simulink model "DC_Parameter_estimation_DREM"  (R2022b)
settings: Solver=VariableStepAuto  StartTime=0.0  StopTime=20  RelTol=1e-3
undefined symbols (not defined in the file): alpha_1, alpha_2, alpha_3
settings Model: Creator=asala  LastModifiedBy=asala

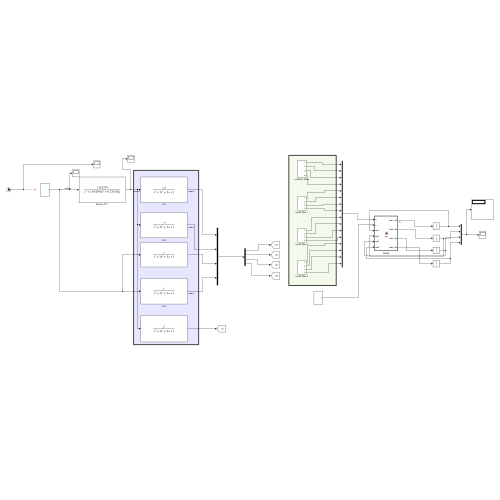
[thumbnail: Simulink's stored preview of the top-level diagram]
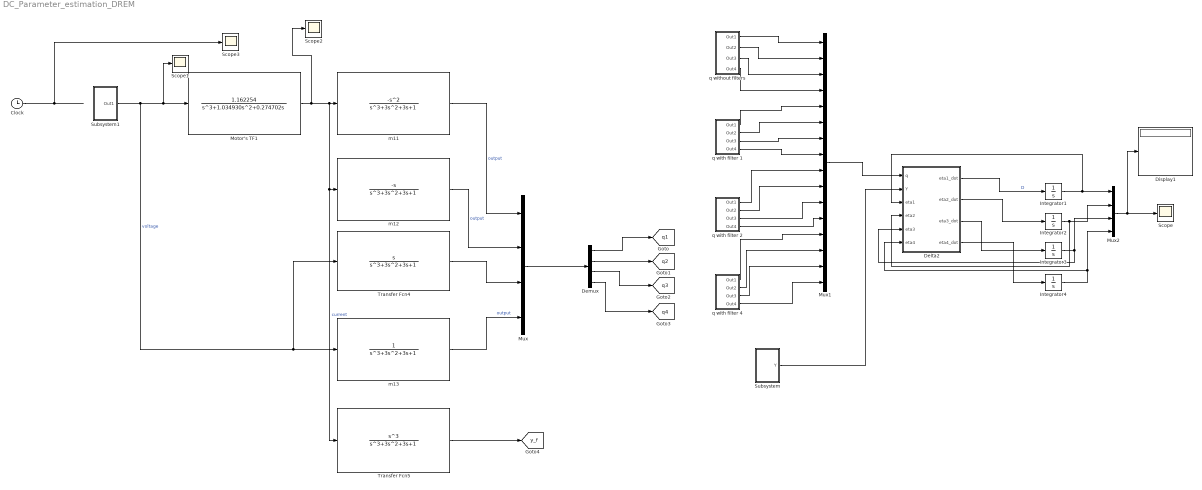
== system DC_Parameter_estimation_DREM ==
  Clock : Clock
  Delta2 : MATLAB Function  TreatAsAtomicUnit=on
  Demux : Demux
  Display1 : Display
  Integrator{1..4} (4 alike) : Integrator
  Motor's TF1 : TransferFcn  Numerator=[1.162254]  Denominator=[1 1.034930 0.274702 0]
  Mux : Mux
  Mux1 : Mux  Inputs=16
  Mux2 : Mux
  Scope{,1..3} (4 alike) : Scope
  Subsystem : Subsystem
  Subsystem1 : Subsystem
  Transfer Fcn4 : TransferFcn  Numerator=[0 1 0]  Denominator=[1, 3, 3, 1]
  Transfer Fcn5 : TransferFcn  Numerator=[1 0 0 0]  Denominator=[1, 3, 3, 1]
  m11 : TransferFcn  Numerator=[-1 0 0]  Denominator=[1, 3, 3, 1]
  m12 : TransferFcn  Numerator=[0 -1 0]  Denominator=[1, 3, 3, 1]
  m13 : TransferFcn  Numerator=[0 0 1]  Denominator=[1, 3, 3, 1]
  q with filter 1 : Subsystem
  q with filter 2 : Subsystem
  q with filter 4 : Subsystem
  q without filters : Subsystem
  tag scope: q1=global, q2=global, q3=global, q4=global, y_f=global
  wires:
  Subsystem1/1(Out1) -> Transfer Fcn4/1, m13/1, Scope1/1, Motor's TF1/1  "voltage"
  Clock/1 -> Scope3/1
  Motor's TF1/1 -> Scope2/1, Transfer Fcn5/1, m12/1, m11/1  "current"
  Demux/3 -> [q3]
  Demux/4 -> [q4]
  Demux/2 -> [q2]
  Demux/1 -> [q1]
  m11/1 -> Mux/1  "output"
  m12/1 -> Mux/2  "output"
  Transfer Fcn4/1 -> Mux/3
  m13/1 -> Mux/4  "output"
  Transfer Fcn5/1 -> [y_f]
  Mux/1 -> Demux/1
  q without filters/1(Out1) -> Mux1/1
  q without filters/2(Out2) -> Mux1/2
  q without filters/3(Out3) -> Mux1/3
  q without filters/4(Out4) -> Mux1/4
  q with filter 1/1(Out1) -> Mux1/5
  q with filter 1/2(Out2) -> Mux1/6
  q with filter 1/3(Out3) -> Mux1/7
  q with filter 1/4(Out4) -> Mux1/8
  q with filter 2/1(Out1) -> Mux1/9
  q with filter 2/2(Out2) -> Mux1/10
  q with filter 2/3(Out3) -> Mux1/11
  q with filter 2/4(Out4) -> Mux1/12
  q with filter 4/1(Out1) -> Mux1/13
  q with filter 4/2(Out2) -> Mux1/14
  q with filter 4/3(Out3) -> Mux1/15
  q with filter 4/4(Out4) -> Mux1/16
  Integrator1/1 -> Delta2/3(eta1), Mux2/1
  Delta2/1(eta1_dot) -> Integrator1/1  "D"
  Delta2/2(eta2_dot) -> Integrator2/1
  Delta2/3(eta3_dot) -> Integrator3/1
  Delta2/4(eta4_dot) -> Integrator4/1
  Integrator4/1 -> Delta2/6(eta4), Mux2/4
  Integrator2/1 -> Delta2/4(eta2), Mux2/2
  Integrator3/1 -> Mux2/3, Delta2/5(eta3)
  Mux1/1 -> Delta2/1(q)
  Subsystem/1(Y) -> Delta2/2(Y)
  Mux2/1 -> Scope/1, Display1/1

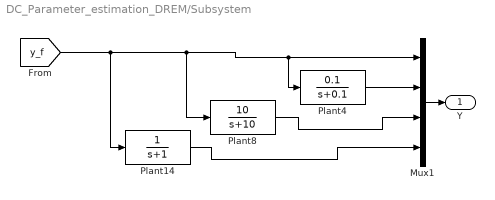
== system DC_Parameter_estimation_DREM/Subsystem ==
  Mux1 : Mux
  Plant14 : TransferFcn  Denominator=[1 1]
  Plant4 : TransferFcn  Numerator=[0.1]  Denominator=[1 0.1]
  Plant8 : TransferFcn  Numerator=[10]  Denominator=[1 10]
  Y : Outport  VectorParamsAs1DForOutWhenUnconnected=off
  wires:
  Mux1/1 -> Y/1
  [y_f] -> Plant14/1, Plant8/1, Plant4/1, Mux1/1
  Plant4/1 -> Mux1/2
  Plant14/1 -> Mux1/4
  Plant8/1 -> Mux1/3

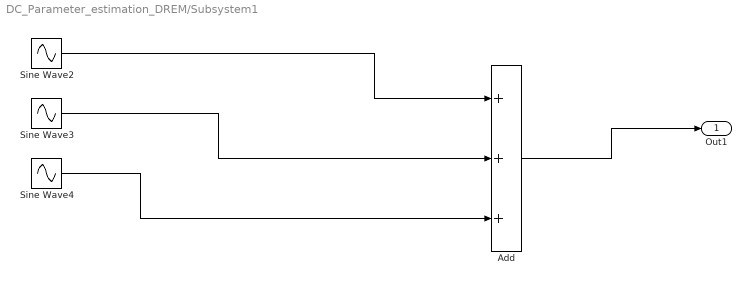
== system DC_Parameter_estimation_DREM/Subsystem1 ==
  Add : Sum  Inputs=+++
  Sine Wave2 : Sin  Amplitude=5  Frequency=2  SampleTime=0
  Sine Wave3 : Sin  Amplitude=2  Frequency=3  SampleTime=0
  Sine Wave4 : Sin  Amplitude=4  SampleTime=0
  Out1 : Outport  VectorParamsAs1DForOutWhenUnconnected=off
  wires:
  Add/1 -> Out1/1
  Sine Wave2/1 -> Add/1
  Sine Wave3/1 -> Add/2
  Sine Wave4/1 -> Add/3

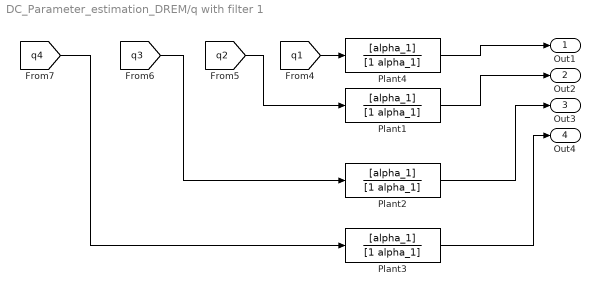
== system DC_Parameter_estimation_DREM/q with filter 1 ==
  Plant{1..4} (4 alike) : TransferFcn  Numerator=[alpha_1]  Denominator=[1 alpha_1]
  Out1 : Outport  VectorParamsAs1DForOutWhenUnconnected=off
  Out2 : Outport  Port=2  VectorParamsAs1DForOutWhenUnconnected=off
  Out3 : Outport  Port=3  VectorParamsAs1DForOutWhenUnconnected=off
  Out4 : Outport  Port=4  VectorParamsAs1DForOutWhenUnconnected=off
  wires:
  [q1] -> Plant4/1
  [q4] -> Plant3/1
  [q3] -> Plant2/1
  Plant2/1 -> Out3/1
  Plant4/1 -> Out1/1
  Plant3/1 -> Out4/1
  [q2] -> Plant1/1
  Plant1/1 -> Out2/1

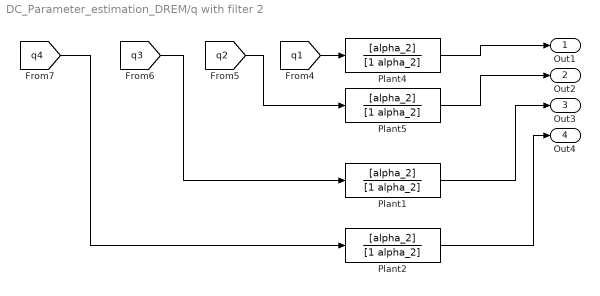
== system DC_Parameter_estimation_DREM/q with filter 2 ==
  Plant{1..2,4..5} (4 alike) : TransferFcn  Numerator=[alpha_2]  Denominator=[1 alpha_2]
  Out1 : Outport  VectorParamsAs1DForOutWhenUnconnected=off
  Out2 : Outport  Port=2  VectorParamsAs1DForOutWhenUnconnected=off
  Out3 : Outport  Port=3  VectorParamsAs1DForOutWhenUnconnected=off
  Out4 : Outport  Port=4  VectorParamsAs1DForOutWhenUnconnected=off
  wires:
  Plant5/1 -> Out2/1
  [q2] -> Plant5/1
  Plant2/1 -> Out4/1
  Plant4/1 -> Out1/1
  Plant1/1 -> Out3/1
  [q3] -> Plant1/1
  [q4] -> Plant2/1
  [q1] -> Plant4/1

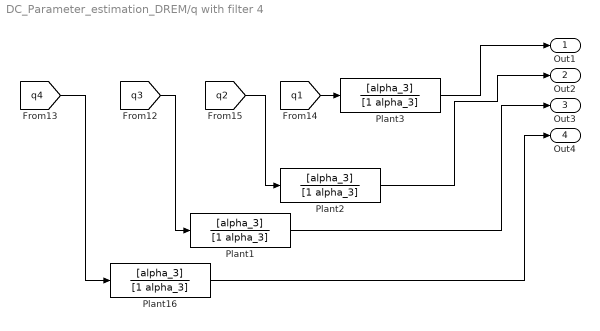
== system DC_Parameter_estimation_DREM/q with filter 4 ==
  Plant{1..3,16} (4 alike) : TransferFcn  Numerator=[alpha_3]  Denominator=[1 alpha_3]
  Out1 : Outport  VectorParamsAs1DForOutWhenUnconnected=off
  Out2 : Outport  Port=2  VectorParamsAs1DForOutWhenUnconnected=off
  Out3 : Outport  Port=3  VectorParamsAs1DForOutWhenUnconnected=off
  Out4 : Outport  Port=4  VectorParamsAs1DForOutWhenUnconnected=off
  wires:
  [q1] -> Plant3/1
  Plant1/1 -> Out3/1
  Plant2/1 -> Out2/1
  [q2] -> Plant2/1
  Plant16/1 -> Out4/1
  Plant3/1 -> Out1/1
  [q4] -> Plant16/1
  [q3] -> Plant1/1

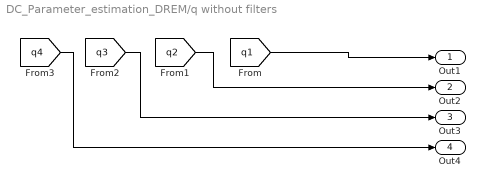
== system DC_Parameter_estimation_DREM/q without filters ==
  Out1 : Outport  VectorParamsAs1DForOutWhenUnconnected=off
  Out2 : Outport  Port=2  VectorParamsAs1DForOutWhenUnconnected=off
  Out3 : Outport  Port=3  VectorParamsAs1DForOutWhenUnconnected=off
  Out4 : Outport  Port=4  VectorParamsAs1DForOutWhenUnconnected=off
  wires:
  [q2] -> Out2/1
  [q4] -> Out4/1
  [q3] -> Out3/1
  [q1] -> Out1/1

== matlab function DC_Parameter_estimation_DREM/Delta2 ==
  data: q input; eta1_dot output; Y input; eta1 input; eta2 input; eta3 input; eta4 input; eta2_dot output; eta3_dot output; eta4_dot output
function [eta1_dot, eta2_dot, eta3_dot, eta4_dot] = fcn(q, Y, eta1, eta2, eta3, eta4)
gamma1=1000;
gamma2=1000;
gamma3=1000;
gamma4=1000;

q11=q(1);
q12=q(2);
q13=q(3);
q14=q(4);
q21=q(5);
q22=q(6);
q23=q(7);
q24=q(8);
q31=q(9);
q32=q(10);
q33=q(11);
q34=q(12);
q41=q(13);
q42=q(14);
q43=q(15);
q44=q(16);

y1=Y(1);
y2=Y(2);
y3=Y(3);
y4=Y(4);

zeta1= y3*(q12*q23*q44 - q12*q24*q43 - q13*q22*q44 + q13*q24*q42 + q14*q22*q43 - q14*q23*q42) - y4*(q12*q23*q34 - q12*q24*q33 - q13*q22*q34 + q13*q24*q32 + q14*q22*q33 - q14*q23*q32) - y2*(q12*q33*q44 - q12*q34*q43 - q13*q32*q44 + q13*q34*q42 + q14*q32*q43 - q14*q33*q42) + y1*(q22*q33*q44 - q22*q34*q43 - q23*q32*q44 + q23*q34*q42 + q24*q32*q43 - q24*q33*q42);
zeta2= y4*(q11*q23*q34 - q11*q24*q33 - q13*q21*q34 + q13*q24*q31 + q14*q21*q33 - q14*q23*q31) - y3*(q11*q23*q44 - q11*q24*q43 - q13*q21*q44 + q13*q24*q41 + q14*q21*q43 - q14*q23*q41) + y2*(q11*q33*q44 - q11*q34*q43 - q13*q31*q44 + q13*q34*q41 + q14*q31*q43 - q14*q33*q41) - y1*(q21*q33*q44 - q21*q34*q43 - q23*q31*q44 + q23*q34*q41 + q24*q31*q43 - q24*q33*q41);
zeta3= y3*(q11*q22*q44 - q11*q24*q42 - q12*q21*q44 + q12*q24*q41 + q14*q21*q42 - q14*q22*q41) - y4*(q11*q22*q34 - q11*q24*q32 - q12*q21*q34 + q12*q24*q31 + q14*q21*q32 - q14*q22*q31) - y2*(q11*q32*q44 - q11*q34*q42 - q12*q31*q44 + q12*q34*q41 + q14*q31*q42 - q14*q32*q41) + y1*(q21*q32*q44 - q21*q34*q42 - q22*q31*q44 + q22*q34*q41 + q24*q31*q42 - q24*q32*q41);
zeta4= y4*(q11*q22*q33 - q11*q23*q32 - q12*q21*q33 + q12*q23*q31 + q13*q21*q32 - q13*q22*q31) - y3*(q11*q22*q43 - q11*q23*q42 - q12*q21*q43 + q12*q23*q41 + q13*q21*q42 - q13*q22*q41) + y2*(q11*q32*q43 - q11*q33*q42 - q12*q31*q43 + q12*q33*q41 + q13*q31*q42 - q13*q32*q41) - y1*(q21*q32*q43 - q21*q33*q42 - q22*q31*q43 + q22*q33*q41 + q23*q31*q42 - q23*q32*q41);



phi=q11*q22*q33*q44 - q11*q22*q34*q43 - q11*q23*q32*q44 + q11*q23*q34*q42 + q11*q24*q32*q43 - q11*q24*q33*q42 - q12*q21*q33*q44 + q12*q21*q34*q43 + q12*q23*q31*q44 - q12*q23*q34*q41 - q12*q24*q31*q43 + q12*q24*q33*q41 + q13*q21*q32*q44 - q13*q21*q34*q42 - q13*q22*q31*q44 + q13*q22*q34*q41 + q13*q24*q31*q42 - q13*q24*q32*q41 - q14*q21*q32*q43 + q14*q21*q33*q42 + q14*q22*q31*q43 - q14*q22*q33*q41 - q14*q23*q31*q42 + q14*q23*q32*q41;


eta1_dot=gamma1*(zeta1*phi-phi*phi*eta1);
eta2_dot=gamma2*(zeta2*phi-phi*phi*eta2);
eta3_dot=gamma3*(zeta3*phi-phi*phi*eta3);
eta4_dot=gamma4*(zeta4*phi-phi*phi*eta4);
